simulink subsystem "MergeActuationSignals"  (R2024a)
settings: Solver=VariableStepAuto  StartTime=0.0  StopTime=10.0  RelTol=1e-3
undefined symbols (not defined in the file): Motor_Rotationals, Motor_Translationals, Transmission_Rotationals, Transmission_Translationals
settings Model: DataDictionary=neck_mk3.sldd  EnableAccessToBaseWorkspace=off  Creator=upattacini  LastModifiedBy=upattacini

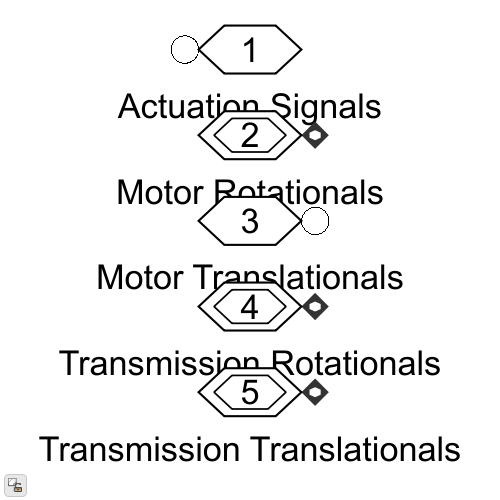
[thumbnail: Simulink's stored preview of the top-level diagram]
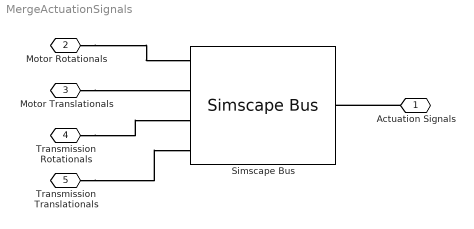
== system MergeActuationSignals ==
  Simscape Bus : SimscapeBus  HierarchyStrings=Motor_Rotationals;Motor_Translationals;Transmission_Rotationals;Transmission_Translationals  ConnectionType=Bus: Physical_Actuation
  Actuation Signals : PMIOPort  Side=Right  ConnectionType=Bus: Physical_Actuation
  Motor Rotationals : PMIOPort  Port=2  Side=Left  ConnectionType=Bus: Physical_MotorRotationals
  Motor Translationals : PMIOPort  Port=3  Side=Left  ConnectionType=Bus: Physical_MotorTranslationals
  Transmission Rotationals : PMIOPort  Port=4  Side=Left  ConnectionType=Bus: Physical_TransmissionRotationals
  Transmission Translationals : PMIOPort  Port=5  Side=Left  ConnectionType=Bus: Physical_TransmissionTranslationals
  connections:
  Actuation Signals/RConn1 -- Simscape Bus/RConn1
  Motor Rotationals/RConn1 -- Simscape Bus/LConn1
  Motor Translationals/RConn1 -- Simscape Bus/LConn2
  Transmission Rotationals/RConn1 -- Simscape Bus/LConn3
  Transmission Translationals/RConn1 -- Simscape Bus/LConn4
